simulink model "BLDCmotorControl_FOC_R2017b"  (R2025a)
settings: Solver=FixedStepDiscrete  StartTime=0  StopTime=1  FixedStep=Ts  MaxStep=1e-6  RelTol=1e-6  AbsTol=1e-6  EnableMultiTasking=on
PreLoadFcn:
  | addpath(genpath('01_Libraries'));
  | addpath(genpath('02_Figures'));
InitFcn:
  | init_model;
undefined symbols (not defined in the file): a_elecAngle, a_elecPeriod, a_phaAdv_M1, b_DCLinkCurrAvail, b_phaAdvEna, b_selPhaABCurrMeas, cf_speedCoef, CTRL_COMM, DiscIntNeverNeededParam, Down, DWORK0, DWORK1, DWORK2, DWORK3, dz_counterHi, dz_counterLo, i_thresOutlier, Kb_Id, Kb_Iq, Kb_n, Ki_Id, Ki_Iq, Ki_n, Kp_Id, Kp_Iq, Kp_n, n_commAcvLo, n_commDeacvHi, n_motPhaAdvEna, r_commDCDeacv, r_sin_M1, r_whl, res_elecAngle, Ts, Ts_ctrl, Up, V_circleLim_M1, V_max, V_min, vec_hallToPos, z_commutMap_M1, z_ctrlTypSel, z_maxCntRst
libraries: eePwmGenerator x7, BLDC_controller_Lib x6, simulink x5, spsControlledVoltageSourceLib x1, spsCurrentMeasurementLib x1, spsPermanentMagnetSynchronousMachineLib x1, spsUniversalBridgeLib x1, spsVoltageMeasurementLib x1, spspowerguiLib x1, SignalEditorBlockLib x1
(part 3 of 3)

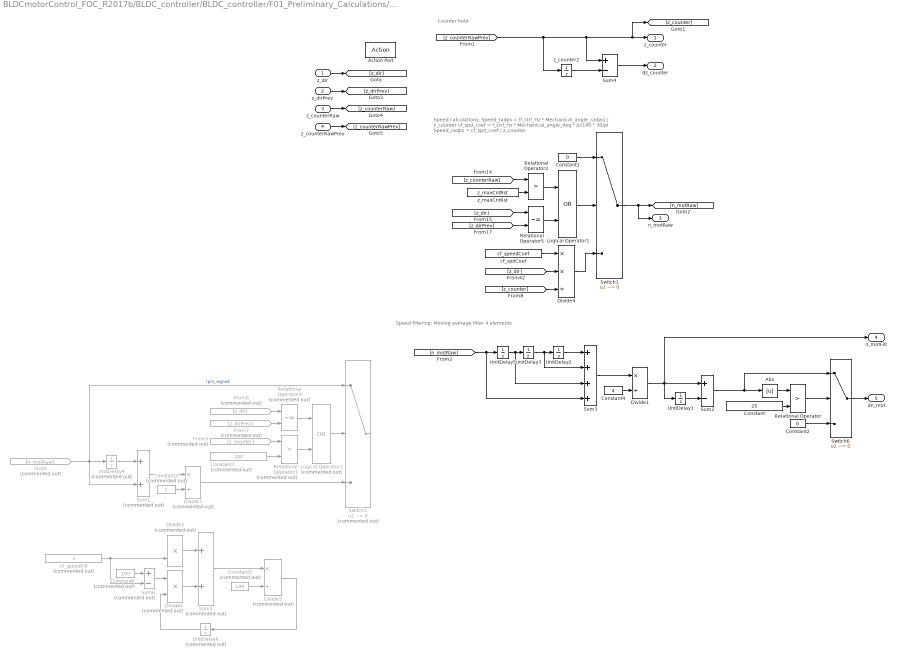
== system BLDCmotorControl_FOC_R2017b/BLDC_controller/BLDC_controller/F01_Preliminary_Calculations/F01_04_Speed_Calculation/Motor_Speed_Calculation ==
  note: Speed calculations:
      | Speed_radps = (f_ctrl_Hz * Mechanical_angle_radps) / z_counter
      | cf_spd_coef = f_ctrl_Hz * Mechanical_angle_deg * pi/180 * 30/pi
      | Speed_radps = cf_spd_coef / z_counter
  note: Speed filtering: Moving average filter 4 elements
  note: Counter hold
  z_dir : Inport
  z_dirPrev : Inport  Port=2
  z_counterRaw : Inport  Port=3
  z_counterRawPrev : Inport  Port=4
  Action Port : ActionPort  ActionPortLabel=if { }
  Abs : Abs  SaturateOnIntegerOverflow=off
  Constant : Constant  Value=25  OutDataTypeStr=Inherit: Inherit via back propagation
  Constant1 : Constant  Value=0  OutDataTypeStr=Inherit: Inherit via back propagation
  Constant2 : Constant  Value=0  OutDataTypeStr=Inherit: Inherit via back propagation
  Constant3 : Constant  Commented=on  Value=2  OutDataTypeStr=Inherit: Inherit via back propagation
  Constant4 : Constant  Value=4  OutDataTypeStr=Inherit: Inherit via back propagation
  Constant5 : Constant  Commented=on  Value=100  OutDataTypeStr=Inherit: Inherit via back propagation
  Constant6 : Constant  Commented=on  Value=100  OutDataTypeStr=Inherit: Inherit via back propagation
  Constant7 : Constant  Commented=on  Value=200  OutDataTypeStr=Inherit: Inherit via back propagation
  Divide1 : Product  Inputs=*/  RndMeth=Simplest
  Divide2 : Product  Commented=on  Inputs=**  RndMeth=Simplest  OutDataTypeStr=Inherit: Same as first input
  Divide3 : Product  Commented=on  Inputs=*/  RndMeth=Simplest
  Divide4 : Product  Inputs=**/  RndMeth=Simplest  OutDataTypeStr=Inherit: Same as first input
  Divide5 : Product  Commented=on  Inputs=*/  RndMeth=Simplest  OutDataTypeStr=Inherit: Same as first input
  Divide6 : Product  Commented=on  Inputs=**  RndMeth=Simplest  OutDataTypeStr=Inherit: Same as first input
  From : From  Commented=on  GotoTag=n_motRaw
  From5 : From  Commented=on  GotoTag=z_counter
  From6 : From  Commented=on  GotoTag=z_dir
  From7 : From  Commented=on  GotoTag=z_dirPrev
  Logical Operator1 : Logic  Operator=OR  AllPortsSameDT=off  OutDataTypeStr=boolean
  Logical Operator2 : Logic  Commented=on  Operator=OR  AllPortsSameDT=off  OutDataTypeStr=boolean
  Relational Operator : RelationalOperator  Operator=>  OutDataTypeStr=boolean  InputSameDT=off
  Relational Operator2 : RelationalOperator  Operator=>  OutDataTypeStr=boolean  RndMeth=Simplest  InputSameDT=off
  Relational Operator3 : RelationalOperator  Commented=on  Operator=>  OutDataTypeStr=boolean  InputSameDT=off
  Relational Operator4 : RelationalOperator  Commented=on  Operator=~=  OutDataTypeStr=boolean  RndMeth=Simplest  InputSameDT=off
  Relational Operator5 : RelationalOperator  Operator=~=  OutDataTypeStr=boolean  RndMeth=Simplest  InputSameDT=off
  Sum1 : Sum  Commented=on  InputSameDT=on  RndMeth=Simplest
  Sum2 : Sum  Inputs=+-  InputSameDT=on  RndMeth=Simplest  OutDataTypeStr=Inherit: Same as first input
  Sum3 : Sum  Inputs=++++  InputSameDT=on  RndMeth=Simplest
  Sum4 : Sum  Inputs=+-  InputSameDT=on  RndMeth=Simplest  OutDataTypeStr=Inherit: Same as first input
  Sum5 : Sum  Commented=on  InputSameDT=on  RndMeth=Simplest  OutDataTypeStr=Inherit: Same as first input
  Sum6 : Sum  Commented=on  Inputs=+-  InputSameDT=on  RndMeth=Simplest  OutDataTypeStr=Inherit: Same as first input
  Switch1 : Switch  Criteria=u2 ~= 0  OutDataTypeStr=Inherit: Inherit via back propagation  RndMeth=Zero  SaturateOnIntegerOverflow=off  InputSameDT=off
  Switch3 : Switch  Commented=on  Criteria=u2 ~= 0  OutDataTypeStr=Inherit: Inherit via back propagation  RndMeth=Zero  SaturateOnIntegerOverflow=off  InputSameDT=off
  Switch6 : Switch  Tag=struct('comment',struct('text','','placement',1),'logdata',struct('maxnumvals',inf,'plotchannels',[],'loggingmode',3,'channels',1),'output',struct('variable','','description','','name','$S_$B','width',1,'address','','max',NaN,'min',NaN,'class','default','type','CONTINUOUS','scaling','','lsb',1,'offset',0,'arb',0,'freeze',1,'unit','','autoscalingmode',1,'lowerheadroom',1,'upperheadroom',1,'headroomunit','bit','keepdatatype',1,'checkmin',0,'checkmax',0,'castoutput',0,'show',0),'threshold',struct('variable','','description','','name','$S_$B_threshold','width',1,'address','','max',NaN,'min',NaN,'class','default','type','CONTINUOUS','scaling','','lsb',1,'offset',0,'arb',0,'freeze',1,'unit','','keepdatatype',1,'value','0','scalar',0,'criteria',3),'scalingvalid',0,'date',733087.49614628474,'inheritscaling',0)  Criteria=u2 ~= 0
      settings: AttributesFormatString=threshold=%<threshold>\nCriteria : %<Criteria>
  UnitDelay{1..3,5} (4 alike) : UnitDelay  SampleTime=-1  HasFrameUpgradeWarning=on
  UnitDelay4 : UnitDelay  Commented=on  SampleTime=-1  HasFrameUpgradeWarning=on
  UnitDelay6 : UnitDelay  Commented=on  SampleTime=-1  HasFrameUpgradeWarning=on
  cf_spdCoef : Constant  Value=cf_speedCoef  OutDataTypeStr=int32
  cf_speedFilt : Constant  Commented=on  Value=3  OutDataTypeStr=int32
  z_counter2 : UnitDelay  InitialCondition=z_maxCntRst  SampleTime=-1  HasFrameUpgradeWarning=on
  z_maxCntRst : Constant  Value=z_maxCntRst  OutDataTypeStr=Inherit: Inherit via back propagation
  z_counter : Outport  InitialOutput=z_maxCntRst  VectorParamsAs1DForOutWhenUnconnected=off
  dz_counter : Outport  Port=2  VectorParamsAs1DForOutWhenUnconnected=off
  n_motRaw : Outport  Port=3  VectorParamsAs1DForOutWhenUnconnected=off
  n_motFilt : Outport  Port=4  VectorParamsAs1DForOutWhenUnconnected=off
  dn_mot : Outport  Port=5  VectorParamsAs1DForOutWhenUnconnected=off
  wires:
  [z_counterRawPrev] -> z_counter2/1, [z_counter], z_counter/1, Sum4/1
  z_counter2/1 -> Sum4/2
  [z_counter] -> Divide4/3
  [z_dir] -> Divide4/2
  cf_spdCoef/1 -> Divide4/1
  z_dir/1 -> [z_dir]
  From/1 -> Switch3/1, Sum1/2, UnitDelay4/1  "rpm_signed"
  UnitDelay4/1 -> Sum1/1
  Sum1/1 -> Divide3/1
  Constant3/1 -> Divide3/2
  [z_dirPrev] -> Relational Operator5/2
  Relational Operator2/1 -> Logical Operator1/1
  Logical Operator1/1 -> Switch1/2
  Relational Operator5/1 -> Logical Operator1/2
  Constant1/1 -> Switch1/1
  z_maxCntRst/1 -> Relational Operator2/2
  [z_counterRaw] -> Relational Operator2/1
  [z_dir] -> Relational Operator5/1
  z_counterRaw/1 -> [z_counterRaw]
  z_dirPrev/1 -> [z_dirPrev]
  z_counterRawPrev/1 -> [z_counterRawPrev]
  UnitDelay1/1 -> Sum2/2
  Relational Operator/1 -> Switch6/2
  Constant2/1 -> Switch6/3
  Abs/1 -> Relational Operator/1
  Constant/1 -> Relational Operator/2
  Switch1/1 -> n_motRaw/1, [n_motRaw]
  Divide4/1 -> Switch1/3
  Sum4/1 -> dz_counter/1
  From5/1 -> Relational Operator3/1
  Constant7/1 -> Relational Operator3/2
  Logical Operator2/1 -> Switch3/2
  Relational Operator3/1 -> Logical Operator2/2
  From6/1 -> Relational Operator4/1
  From7/1 -> Relational Operator4/2
  Relational Operator4/1 -> Logical Operator2/1
  Divide3/1 -> Switch3/3
  Divide1/1 -> n_motFilt/1, Sum2/1, UnitDelay1/1
  Constant4/1 -> Divide1/2
  Sum3/1 -> Divide1/1
  UnitDelay2/1 -> Sum3/1
  UnitDelay3/1 -> Sum3/2, UnitDelay2/1
  UnitDelay5/1 -> Sum3/3, UnitDelay3/1
  [n_motRaw] -> Sum3/4, UnitDelay5/1
  UnitDelay6/1 -> Divide6/2
  Sum5/1 -> Divide5/1
  Constant6/1 -> Sum6/1
  Divide6/1 -> Sum5/2
  Sum6/1 -> Divide6/1
  cf_speedFilt/1 -> Divide2/2, Sum6/2
  Constant5/1 -> Divide5/2
  Divide5/1 -> UnitDelay6/1
  Divide2/1 -> Sum5/1
  Switch6/1 -> dn_mot/1
  Sum2/1 -> Switch6/1, Abs/1

== system BLDCmotorControl_FOC_R2017b/BLDC_controller/BLDC_controller/F03_Field_Oriented_Control/Clarke_Transform/Clarke_PhasesAB ==
  note: Clarke Transform:
      | i_alpha = i_phaA
      | i_beta = ((1/sqrt(3))*i_phaA + (2/sqrt(3))*i_phaB)
  i_phaA : Inport
  i_phaB : Inport  Port=2
  Action Port : ActionPort  ActionPortLabel=if { }
  Gain1 : Gain  Tag=struct('comment',struct('text','','placement',1),'logdata',struct('maxnumvals',inf,'plotchannels',[],'loggingmode',3,'channels',1),'output',struct('variable','','description','','name','$S_$B','width',1,'address','','max',NaN,'min',NaN,'class','default','type','CONTINUOUS','scaling','','lsb',1,'offset',0,'arb',0,'freeze',1,'unit','','autoscalingmode',1,'lowerheadroom',1,'upperheadroom',1,'headroomunit','bit','keepdatatype',1,'checkmin',0,'checkmax',0,'castoutput',0,'show',0),'gain',struct('variable','','description','','name','$S_$B_gain','width',1,'address','','max',NaN,'min',NaN,'class','default','type','CONTINUOUS','scaling','','lsb',1,'offset',0,'arb',0,'freeze',1,'unit','','keepdatatype',1,'value','1','scalar',0,'tolerance',1),'scalingvalid',0,'date',730486)  Gain=2/sqrt(3)  RndMeth=Zero
  Gain3 : Gain  Tag=struct('comment',struct('text','','placement',1),'logdata',struct('maxnumvals',inf,'plotchannels',[],'loggingmode',3,'channels',1),'output',struct('variable','','description','','name','$S_$B','width',1,'address','','max',NaN,'min',NaN,'class','default','type','CONTINUOUS','scaling','','lsb',1,'offset',0,'arb',0,'freeze',1,'unit','','autoscalingmode',1,'lowerheadroom',1,'upperheadroom',1,'headroomunit','bit','keepdatatype',1,'checkmin',0,'checkmax',0,'castoutput',0,'show',0),'gain',struct('variable','','description','','name','$S_$B_gain','width',1,'address','','max',NaN,'min',NaN,'class','default','type','CONTINUOUS','scaling','','lsb',1,'offset',0,'arb',0,'freeze',1,'unit','','keepdatatype',1,'value','1','scalar',0,'tolerance',1),'scalingvalid',0,'date',730486)  Gain=1/sqrt(3)  RndMeth=Zero
  Sum6 : Sum  RndMeth=Simplest
  for_merge : Gain  Tag=struct('comment',struct('text','','placement',1),'logdata',struct('maxnumvals',inf,'plotchannels',[],'loggingmode',3,'channels',1),'output',struct('variable','','description','','name','$S_$B','width',1,'address','','max',NaN,'min',NaN,'class','default','type','CONTINUOUS','scaling','','lsb',1,'offset',0,'arb',0,'freeze',1,'unit','','autoscalingmode',1,'lowerheadroom',1,'upperheadroom',1,'headroomunit','bit','keepdatatype',1,'checkmin',0,'checkmax',0,'castoutput',0,'show',0),'gain',struct('variable','','description','','name','$S_$B_gain','width',1,'address','','max',NaN,'min',NaN,'class','default','type','CONTINUOUS','scaling','','lsb',1,'offset',0,'arb',0,'freeze',1,'unit','','keepdatatype',1,'value','1','scalar',0,'tolerance',1),'scalingvalid',0,'date',730486)  RndMeth=Zero
  i_alphaAB : Outport  VectorParamsAs1DForOutWhenUnconnected=off
  i_betaAB : Outport  Port=2  VectorParamsAs1DForOutWhenUnconnected=off
  wires:
  i_phaB/1 -> [i_phaB]
  i_phaA/1 -> [i_phaA]
  [i_phaB] -> Gain1/1
  [i_phaA] -> for_merge/1, Gain3/1
  Gain3/1 -> Sum6/1
  Sum6/1 -> i_betaAB/1  "beta"
  Gain1/1 -> Sum6/2
  for_merge/1 -> i_alphaAB/1

== system BLDCmotorControl_FOC_R2017b/BLDC_controller/BLDC_controller/F03_Field_Oriented_Control/Clarke_Transform/Clarke_PhasesBC ==
  note: Clarke Transform:
      | i_alpha = - i_phaB - i_phaC
      | i_beta = (1/sqrt(3)) * (i_phaB - i_phaC)
  i_phaB : Inport
  i_phaC : Inport  Port=2
  Action Port : ActionPort  ActionPortLabel=else { }
  Gain2 : Gain  Tag=struct('comment',struct('text','','placement',1),'logdata',struct('maxnumvals',inf,'plotchannels',[],'loggingmode',3,'channels',1),'output',struct('variable','','description','','name','$S_$B','width',1,'address','','max',NaN,'min',NaN,'class','default','type','CONTINUOUS','scaling','','lsb',1,'offset',0,'arb',0,'freeze',1,'unit','','autoscalingmode',1,'lowerheadroom',1,'upperheadroom',1,'headroomunit','bit','keepdatatype',1,'checkmin',0,'checkmax',0,'castoutput',0,'show',0),'gain',struct('variable','','description','','name','$S_$B_gain','width',1,'address','','max',NaN,'min',NaN,'class','default','type','CONTINUOUS','scaling','','lsb',1,'offset',0,'arb',0,'freeze',1,'unit','','keepdatatype',1,'value','1','scalar',0,'tolerance',1),'scalingvalid',0,'date',730486)  Gain=1/sqrt(3)  RndMeth=Zero
  Sum1 : Sum  Inputs=--  RndMeth=Simplest
  Sum2 : Sum  Inputs=+-  RndMeth=Simplest
  i_alphaBC : Outport  VectorParamsAs1DForOutWhenUnconnected=off
  i_betaBC : Outport  Port=2  VectorParamsAs1DForOutWhenUnconnected=off
  wires:
  [i_phaC] -> Sum1/2
  [i_phaB] -> Sum1/1
  [i_phaC] -> Sum2/2
  Gain2/1 -> i_betaBC/1
  Sum2/1 -> Gain2/1
  [i_phaB] -> Sum2/1
  Sum1/1 -> i_alphaBC/1
  i_phaB/1 -> [i_phaB]
  i_phaC/1 -> [i_phaC]

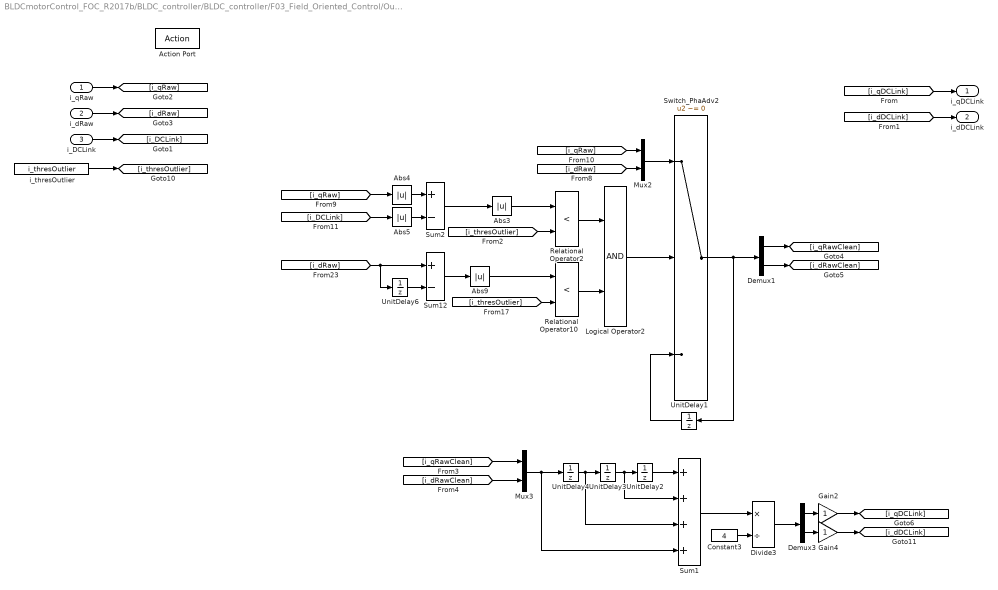
== system BLDCmotorControl_FOC_R2017b/BLDC_controller/BLDC_controller/F03_Field_Oriented_Control/Outliers_Removal/DCLink_Current_Available ==
  i_qRaw : Inport
  i_dRaw : Inport  Port=2
  i_DCLink : Inport  Port=3
  Action Port : ActionPort  ActionPortLabel=if { }
  Abs{3..5,9} (4 alike) : Abs  SaturateOnIntegerOverflow=off
  Constant3 : Constant  Value=4  OutDataTypeStr=Inherit: Inherit via back propagation
  Demux1 : Demux  Outputs=2
  Demux3 : Demux  Outputs=2
  Divide3 : Product  Inputs=*/  RndMeth=Simplest
  Gain2 : Gain  Tag=struct('comment',struct('text','','placement',1),'logdata',struct('maxnumvals',inf,'plotchannels',[],'loggingmode',3,'channels',1),'output',struct('variable','','description','','name','$S_$B','width',1,'address','','max',NaN,'min',NaN,'class','default','type','CONTINUOUS','scaling','','lsb',1,'offset',0,'arb',0,'freeze',1,'unit','','autoscalingmode',1,'lowerheadroom',1,'upperheadroom',1,'headroomunit','bit','keepdatatype',1,'checkmin',0,'checkmax',0,'castoutput',0,'show',0),'gain',struct('variable','','description','','name','$S_$B_gain','width',1,'address','','max',NaN,'min',NaN,'class','default','type','CONTINUOUS','scaling','','lsb',1,'offset',0,'arb',0,'freeze',1,'unit','','keepdatatype',1,'value','1','scalar',0,'tolerance',1),'scalingvalid',0,'date',730486)  RndMeth=Zero  SaturateOnIntegerOverflow=on  OutDataTypeStr=Inherit: Same as input  ParamDataTypeStr=Inherit: Same as input
  Gain4 : Gain  Tag=struct('comment',struct('text','','placement',1),'logdata',struct('maxnumvals',inf,'plotchannels',[],'loggingmode',3,'channels',1),'output',struct('variable','','description','','name','$S_$B','width',1,'address','','max',NaN,'min',NaN,'class','default','type','CONTINUOUS','scaling','','lsb',1,'offset',0,'arb',0,'freeze',1,'unit','','autoscalingmode',1,'lowerheadroom',1,'upperheadroom',1,'headroomunit','bit','keepdatatype',1,'checkmin',0,'checkmax',0,'castoutput',0,'show',0),'gain',struct('variable','','description','','name','$S_$B_gain','width',1,'address','','max',NaN,'min',NaN,'class','default','type','CONTINUOUS','scaling','','lsb',1,'offset',0,'arb',0,'freeze',1,'unit','','keepdatatype',1,'value','1','scalar',0,'tolerance',1),'scalingvalid',0,'date',730486)  RndMeth=Zero  SaturateOnIntegerOverflow=on  OutDataTypeStr=Inherit: Same as input  ParamDataTypeStr=Inherit: Same as input
  Logical Operator2 : Logic  AllPortsSameDT=off  OutDataTypeStr=boolean
  Mux2 : Mux  Inputs=2
  Mux3 : Mux  Inputs=2
  Relational Operator10 : RelationalOperator  Operator=<  OutDataTypeStr=boolean  RndMeth=Simplest  InputSameDT=off
  Relational Operator2 : RelationalOperator  Operator=<  OutDataTypeStr=boolean  RndMeth=Simplest  InputSameDT=off
  Sum1 : Sum  Inputs=++++  InputSameDT=on  RndMeth=Simplest
  Sum12 : Sum  Inputs=+-  RndMeth=Simplest
  Sum2 : Sum  Inputs=+-  RndMeth=Simplest
  Switch_PhaAdv2 : Switch  Criteria=u2 ~= 0  OutDataTypeStr=Inherit: Inherit via back propagation  RndMeth=Zero  SaturateOnIntegerOverflow=off  InputSameDT=off
  UnitDelay{1..4,6} (5 alike) : UnitDelay  SampleTime=-1  HasFrameUpgradeWarning=on
  i_thresOutlier : Constant  Value=i_thresOutlier  OutDataTypeStr=Inherit: Inherit via back propagation
  i_qDCLink : Outport  VectorParamsAs1DForOutWhenUnconnected=off
  i_dDCLink : Outport  Port=2  VectorParamsAs1DForOutWhenUnconnected=off
  wires:
  [i_dDCLink] -> i_dDCLink/1
  i_qRaw/1 -> [i_qRaw]
  [i_qDCLink] -> i_qDCLink/1
  i_dRaw/1 -> [i_dRaw]
  i_DCLink/1 -> [i_DCLink]
  Switch_PhaAdv2/1 -> Demux1/1, UnitDelay1/1
  Mux2/1 -> Switch_PhaAdv2/1
  Logical Operator2/1 -> Switch_PhaAdv2/2
  [i_DCLink] -> Abs5/1
  UnitDelay6/1 -> Sum12/2
  Demux1/1 -> [i_qRawClean]
  [i_thresOutlier] -> Relational Operator2/2
  Relational Operator10/1 -> Logical Operator2/2
  [i_dRaw] -> Mux2/2
  Abs9/1 -> Relational Operator10/1
  [i_thresOutlier] -> Relational Operator10/2
  Abs5/1 -> Sum2/2
  [i_dRaw] -> UnitDelay6/1, Sum12/1
  Abs3/1 -> Relational Operator2/1
  Demux1/2 -> [i_dRawClean]
  UnitDelay1/1 -> Switch_PhaAdv2/3
  [i_qRaw] -> Abs4/1
  [i_qRaw] -> Mux2/1
  Abs4/1 -> Sum2/1
  Relational Operator2/1 -> Logical Operator2/1
  Sum2/1 -> Abs3/1
  Sum12/1 -> Abs9/1
  Demux3/2 -> Gain4/1
  Gain2/1 -> [i_qDCLink]
  Divide3/1 -> Demux3/1
  Mux3/1 -> Sum1/4, UnitDelay4/1
  Gain4/1 -> [i_dDCLink]
  UnitDelay4/1 -> Sum1/3, UnitDelay3/1
  [i_qRawClean] -> Mux3/1
  Sum1/1 -> Divide3/1
  UnitDelay3/1 -> Sum1/2, UnitDelay2/1
  Constant3/1 -> Divide3/2
  UnitDelay2/1 -> Sum1/1
  Demux3/1 -> Gain2/1
  [i_dRawClean] -> Mux3/2
  i_thresOutlier/1 -> [i_thresOutlier]

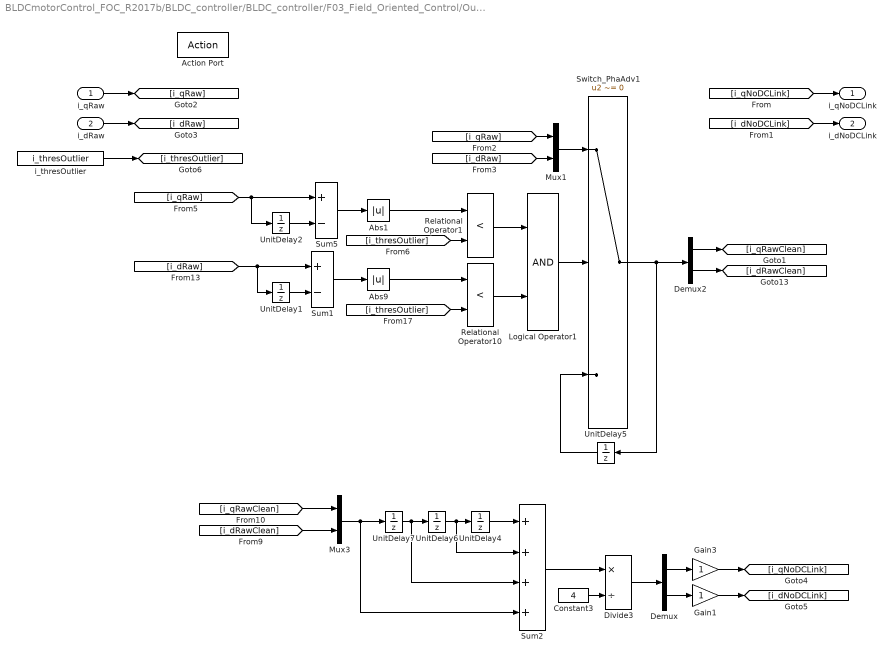
== system BLDCmotorControl_FOC_R2017b/BLDC_controller/BLDC_controller/F03_Field_Oriented_Control/Outliers_Removal/DCLink_Current_Not_Available ==
  i_qRaw : Inport
  i_dRaw : Inport  Port=2
  Action Port : ActionPort  ActionPortLabel=else { }
  Abs1 : Abs  SaturateOnIntegerOverflow=off
  Abs9 : Abs  SaturateOnIntegerOverflow=off
  Constant3 : Constant  Value=4  OutDataTypeStr=Inherit: Inherit via back propagation
  Demux : Demux  Outputs=2
  Demux2 : Demux  Outputs=2
  Divide3 : Product  Inputs=*/  RndMeth=Simplest
  Gain1 : Gain  Tag=struct('comment',struct('text','','placement',1),'logdata',struct('maxnumvals',inf,'plotchannels',[],'loggingmode',3,'channels',1),'output',struct('variable','','description','','name','$S_$B','width',1,'address','','max',NaN,'min',NaN,'class','default','type','CONTINUOUS','scaling','','lsb',1,'offset',0,'arb',0,'freeze',1,'unit','','autoscalingmode',1,'lowerheadroom',1,'upperheadroom',1,'headroomunit','bit','keepdatatype',1,'checkmin',0,'checkmax',0,'castoutput',0,'show',0),'gain',struct('variable','','description','','name','$S_$B_gain','width',1,'address','','max',NaN,'min',NaN,'class','default','type','CONTINUOUS','scaling','','lsb',1,'offset',0,'arb',0,'freeze',1,'unit','','keepdatatype',1,'value','1','scalar',0,'tolerance',1),'scalingvalid',0,'date',730486)  RndMeth=Zero  SaturateOnIntegerOverflow=on  OutDataTypeStr=Inherit: Same as input  ParamDataTypeStr=Inherit: Same as input
  Gain3 : Gain  Tag=struct('comment',struct('text','','placement',1),'logdata',struct('maxnumvals',inf,'plotchannels',[],'loggingmode',3,'channels',1),'output',struct('variable','','description','','name','$S_$B','width',1,'address','','max',NaN,'min',NaN,'class','default','type','CONTINUOUS','scaling','','lsb',1,'offset',0,'arb',0,'freeze',1,'unit','','autoscalingmode',1,'lowerheadroom',1,'upperheadroom',1,'headroomunit','bit','keepdatatype',1,'checkmin',0,'checkmax',0,'castoutput',0,'show',0),'gain',struct('variable','','description','','name','$S_$B_gain','width',1,'address','','max',NaN,'min',NaN,'class','default','type','CONTINUOUS','scaling','','lsb',1,'offset',0,'arb',0,'freeze',1,'unit','','keepdatatype',1,'value','1','scalar',0,'tolerance',1),'scalingvalid',0,'date',730486)  RndMeth=Zero  SaturateOnIntegerOverflow=on  OutDataTypeStr=Inherit: Same as input  ParamDataTypeStr=Inherit: Same as input
  Logical Operator1 : Logic  AllPortsSameDT=off  OutDataTypeStr=boolean
  Mux1 : Mux  Inputs=2
  Mux3 : Mux  Inputs=2
  Relational Operator1 : RelationalOperator  Operator=<  OutDataTypeStr=boolean  RndMeth=Simplest  InputSameDT=off
  Relational Operator10 : RelationalOperator  Operator=<  OutDataTypeStr=boolean  RndMeth=Simplest  InputSameDT=off
  Sum1 : Sum  Inputs=+-  RndMeth=Simplest
  Sum2 : Sum  Inputs=++++  InputSameDT=on  RndMeth=Simplest
  Sum5 : Sum  Inputs=+-  RndMeth=Simplest
  Switch_PhaAdv1 : Switch  Criteria=u2 ~= 0  OutDataTypeStr=Inherit: Inherit via back propagation  RndMeth=Zero  SaturateOnIntegerOverflow=off  InputSameDT=off
  UnitDelay{1..2,4..7} (6 alike) : UnitDelay  SampleTime=-1  HasFrameUpgradeWarning=on
  i_thresOutlier : Constant  Value=i_thresOutlier  OutDataTypeStr=Inherit: Inherit via back propagation
  i_qNoDCLink : Outport  VectorParamsAs1DForOutWhenUnconnected=off
  i_dNoDCLink : Outport  Port=2  VectorParamsAs1DForOutWhenUnconnected=off
  wires:
  i_qRaw/1 -> [i_qRaw]
  i_dRaw/1 -> [i_dRaw]
  [i_qNoDCLink] -> i_qNoDCLink/1
  [i_dNoDCLink] -> i_dNoDCLink/1
  Logical Operator1/1 -> Switch_PhaAdv1/2
  Constant3/1 -> Divide3/2
  UnitDelay6/1 -> Sum2/2, UnitDelay4/1
  UnitDelay7/1 -> Sum2/3, UnitDelay6/1
  [i_qRawClean] -> Mux3/1
  Sum1/1 -> Abs9/1
  Abs9/1 -> Relational Operator10/1
  [i_dRaw] -> UnitDelay1/1, Sum1/1
  Sum2/1 -> Divide3/1
  [i_thresOutlier] -> Relational Operator10/2
  Divide3/1 -> Demux/1
  Demux2/1 -> [i_qRawClean]
  Demux/1 -> Gain3/1
  Demux2/2 -> [i_dRawClean]
  Relational Operator10/1 -> Logical Operator1/2
  UnitDelay1/1 -> Sum1/2
  Abs1/1 -> Relational Operator1/1
  Gain3/1 -> [i_qNoDCLink]
  [i_qRaw] -> Mux1/1
  Sum5/1 -> Abs1/1
  [i_thresOutlier] -> Relational Operator1/2
  Gain1/1 -> [i_dNoDCLink]
  Mux3/1 -> Sum2/4, UnitDelay7/1
  Mux1/1 -> Switch_PhaAdv1/1
  Switch_PhaAdv1/1 -> Demux2/1, UnitDelay5/1
  UnitDelay4/1 -> Sum2/1
  [i_dRaw] -> Mux1/2
  UnitDelay2/1 -> Sum5/2
  UnitDelay5/1 -> Switch_PhaAdv1/3
  Relational Operator1/1 -> Logical Operator1/1
  [i_qRaw] -> Sum5/1, UnitDelay2/1
  [i_dRawClean] -> Mux3/2
  Demux/2 -> Gain1/1
  i_thresOutlier/1 -> [i_thresOutlier]
